simulink model "observerModel_GVS_MS"  (R2023b)
settings: Solver=ode15s  StartTime=0.0  StopTime=duration  MaxStep=0.02  RelTol=0.02  AbsTol=0.02  EnableMultiTasking=on
values from neighbouring files (symbols this model uses):
  beta1 = s(8)    [Observer_Analysis.m]
  beta2 = s(7)    [Observer_Analysis.m]
  delta_t = time(2) - time (1)    [Observer_Analysis.m]
  df = 1    [Observer_Analysis.m]
  f_oto = 2    [Observer_Analysis.m]
  f_scc = 2    [Observer_Analysis.m]
  f_visO = 0.2    [Observer_Analysis.m]
  f_visV = 2    [Observer_Analysis.m]
  f_visX = 2    [Observer_Analysis.m]
  GG0 = [0 0 -hypo]'    [Observer_Analysis.m]
  IrregDepol = tf(num,den)    [Observer_Analysis.m]
  IrregHyperpol = tf(num,den)    [Observer_Analysis.m]
  IrregSCC2Physical = inv(IrregSCCnf)    [Observer_Analysis.m]
  kaa = -3.2*[1 1 1]'    [Observer_Analysis.m]
  Kea = s(1)^(1/2)*[1 1 1]    [Observer_Analysis.m]
  Kef = s(3)^(1/2)*[1 1 1]    [Observer_Analysis.m]
  Kew = s(2)^(1/2)*[1 1 1]    [Observer_Analysis.m]
  Kfast = s(4)    [Observer_Analysis.m]
  kfg = 4*[1 1 1]'    [Observer_Analysis.m]
  kfw = 8*[1 1 1]'    [Observer_Analysis.m]
  kgvg = 5*[1 1 1]'    [Observer_Analysis.m]
  KLeft = 1-KRight    (= 0.5)    [Observer_Analysis.m]
  KReg = s2(2)    [Observer_Analysis.m]
  KRight = 0.5    [Observer_Analysis.m]
  KS = s2(1)*pi/180    [Observer_Analysis.m]
  kwg = 1*[1 1 1]'    [Observer_Analysis.m]
  kwvw = 10*[1 1 1]'    [Observer_Analysis.m]
  kww = 2.28*[1 1 1]'    [Observer_Analysis.m]
  kxdotva = 0.75*[1 1 1]'    [Observer_Analysis.m]
  kxvv = 0.1*[1 1 1]'    [Observer_Analysis.m]
  LeftSide_CurrentMult = s2(4)    [Observer_Analysis.m]
  ms_exp = s(6)    [Observer_Analysis.m]
  oto_a = 60*[1 1 1]'    [Observer_Analysis.m]
  oto_Ka = 1.3*[1 1 1]'    [Observer_Analysis.m]
  Q0 = [cos(E_angle/2) E(1)*sin(E_angle/2) E(2)*sin(E_angle/2) E(3)*sin(E_angle/2)]'    [Observer_Analysis.m]
  RegDepol = tf(num,den)    [Observer_Analysis.m]
  RegHyperpol = tf(num,den)    [Observer_Analysis.m]
  RegSCC2Physical = inv(RegSCCnf)    [Observer_Analysis.m]
  tau_a = tau_a_value*[1 1 1]'    [Observer_Analysis.m]
  tau_scc = tau_scc_value*[1 1 1]'    [Observer_Analysis.m]
  x_leak = 0.6    [Observer_Analysis.m]
  y_leak = 0.6    [Observer_Analysis.m]
  z_leak = 10    [Observer_Analysis.m]
(part 2 of 3)

== system observerModel_GVS_MS/Motion Sickness Dynamics/Oman 1 ==
  note: Ks = 5, Ts = 600sec, ns = 2
  note: Tf = 60sec, nf = 2
  note: if nf = 2, as Oman has it
  In1 : Inport
  Add1 : Sum
  Product : Product
  Transfer Fcn : TransferFcn  Numerator=[Kfast]  Denominator=[beta1^2 2*df*beta1 1]
  Transfer Fcn2 : TransferFcn  Denominator=[beta2^2 2*beta2 1]
  I(t) : Outport  VectorParamsAs1DForOutWhenUnconnected=off
  F(t) : Outport  Port=2  VectorParamsAs1DForOutWhenUnconnected=off
  S(t) : Outport  Port=3  VectorParamsAs1DForOutWhenUnconnected=off
  wires:
  Add1/1 -> I(t)/1  "I(t)"
  Transfer Fcn2/1 -> S(t)/1, Product/2, Add1/2  "S(t)"
  Transfer Fcn/1 -> Add1/1, F(t)/1  "F(t)"
  In1/1 -> Transfer Fcn2/1, Product/1
  Product/1 -> Transfer Fcn/1

== system observerModel_GVS_MS/Otoliths/X Graviceptor ==
  in_1 : Inport
  Adaptation : TransferFcn  Numerator=[oto_Ka(1)*oto_a(1) 1]  Denominator=[oto_a(1) 1]
  Low Pass Filter : TransferFcn  Denominator=[1/(2*pi*f_oto) 1]
  New Otolith model : TransferFcn  Numerator=[333 33.3]  Denominator="[0.08  5.016 1]"
  Scope{,1..3} (4 alike) : Scope
  X Graviceptor : TransferFcn  Numerator=[oto_Ka(1)*oto_a(1) 1]  Denominator=[oto_a(1)*1/(2*pi*f_oto) (1/(2*pi*f_oto)+oto_a(1)) 1]
  out_1 : Outport  InitialOutput=0
  wires:
  in_1/1 -> Low Pass Filter/1, X Graviceptor/1, Adaptation/1, New Otolith model/1
  Low Pass Filter/1 -> out_1/1, Scope2/1
  X Graviceptor/1 -> Scope/1
  Adaptation/1 -> Scope1/1
  New Otolith model/1 -> Scope3/1

== system observerModel_GVS_MS/Otoliths/Y Graviceptor ==
  in_1 : Inport
  Adaptation : TransferFcn  Numerator=[oto_Ka(2)*oto_a(2) 1]  Denominator=[oto_a(2) 1]
  Low Pass Filter : TransferFcn  Denominator=[1/(2*pi*f_oto) 1]
  New Otolith model : TransferFcn  Numerator=[333 33.3]  Denominator="[0.08  5.016 1]"
  Scope{,1..3} (4 alike) : Scope
  X Graviceptor : TransferFcn  Numerator=[oto_Ka(2)*oto_a(2) 1]  Denominator=[oto_a(2)*1/(2*pi*f_oto) (1/(2*pi*f_oto)+oto_a(2)) 1]
  out_1 : Outport  InitialOutput=0
  wires:
  in_1/1 -> Low Pass Filter/1, X Graviceptor/1, Adaptation/1, New Otolith model/1
  Low Pass Filter/1 -> out_1/1, Scope2/1
  X Graviceptor/1 -> Scope/1
  Adaptation/1 -> Scope1/1
  New Otolith model/1 -> Scope3/1

== system observerModel_GVS_MS/Otoliths/Z Graviceptor ==
  in_1 : Inport
  Adaptation : TransferFcn  Numerator=[oto_Ka(3)*oto_a(3) 1]  Denominator=[oto_a(3) 1]
  Low Pass Filter : TransferFcn  Denominator=[1/(2*pi*f_oto) 1]
  New Otolith model : TransferFcn  Numerator=[333 33.3]  Denominator="[0.08  5.016 1]"
  Scope{,1..3} (4 alike) : Scope
  X Graviceptor : TransferFcn  Numerator=[oto_Ka(3)*oto_a(3) 1]  Denominator=[oto_a(3)*1/(2*pi*f_oto) (1/(2*pi*f_oto)+oto_a(3)) 1]
  out_1 : Outport  InitialOutput=0
  wires:
  Low Pass Filter/1 -> out_1/1, Scope2/1
  X Graviceptor/1 -> Scope/1
  Adaptation/1 -> Scope1/1
  New Otolith model/1 -> Scope3/1
  in_1/1 -> Low Pass Filter/1, X Graviceptor/1, Adaptation/1, New Otolith model/1

== system observerModel_GVS_MS/Quaternion Rotator/Head to Limbic Angular Velocity Transform ==
  omega_head : Inport
  D_Cos : Inport  Port=2
  Gain : Gain  Gain=-1
  Product1 : Product  Multiplication=Matrix(*)  RndMeth=Zero
  Quaternion Integrator1 : Subsystem
  Quaternion to Direction Cosine1 : Subsystem
  Transform Axes : Subsystem
  Transpose : Math  Operator=transpose  SignedPower=on
  R_limbic : Outport
  wires:
  Quaternion Integrator1/1(q) -> Quaternion to Direction Cosine1/1(q)
  Quaternion to Direction Cosine1/1(D_Cos) -> R_limbic/1
  omega_head/1 -> Product1/2
  Transpose/1 -> Product1/1
  D_Cos/1 -> Transpose/1
  Product1/1 -> Transform Axes/1(limbic_cord)
  Transform Axes/1(VR_cord) -> Gain/1
  Gain/1 -> Quaternion Integrator1/1(omega_limbic)

== system observerModel_GVS_MS/Quaternion Rotator/Quaternion Integrator ==
  omega_head : Inport
  Demux1 : Demux
  Gain : Gain  Gain=1/delta_t
  Mux1 : Mux
  delta_q : Subsystem
  q0 : Integrator  InitialCondition=Q0(1)
  q1 : Integrator  InitialCondition=Q0(2)
  q2 : Integrator  InitialCondition=Q0(3)
  q3 : Integrator  InitialCondition=Q0(4)
  q : Outport
  wires:
  Demux1/1 -> q0/1
  q0/1 -> Mux1/1
  Demux1/2 -> q1/1
  q1/1 -> Mux1/2
  Demux1/3 -> q2/1
  q2/1 -> Mux1/3
  Demux1/4 -> q3/1
  q3/1 -> Mux1/4
  Mux1/1 -> delta_q/2(q), q/1
  Gain/1 -> Demux1/1
  delta_q/1(delta_q) -> Gain/1
  omega_head/1 -> delta_q/1(omega)

== system observerModel_GVS_MS/Quaternion Rotator/Quaternion to Direction Cosine ==
  note: A21
  q : Inport
  A1 : Subsystem
  A11 : Subsystem
  A12 : Subsystem
  A13 : Subsystem
  A22 : Subsystem
  A23 : Subsystem
  A31 : Subsystem
  A32 : Subsystem
  A33 : Subsystem
  Mux : Mux  Inputs=9
  Reshape (9) to [3x3] column-major : Reshape  OutputDimensionality=Customize  OutputDimensions=[3,3]
  D_Cos : Outport
  wires:
  A33/1(A33) -> Mux/9
  A32/1(A32) -> Mux/6
  A31/1(A31) -> Mux/3
  A23/1(A23) -> Mux/8
  A22/1(A22) -> Mux/5
  A13/1(A13) -> Mux/7
  A12/1(A12) -> Mux/4
  A11/1(A11) -> Mux/1
  q/1 -> A22/1(q), A1/1(q), A13/1(q), A12/1(q), A11/1(q), A23/1(q), A31/1(q), A32/1(q), A33/1(q)
  Reshape (9) to [3x3] column-major/1 -> D_Cos/1
  A1/1(A21) -> Mux/2
  Mux/1 -> Reshape (9) to [3x3] column-major/1

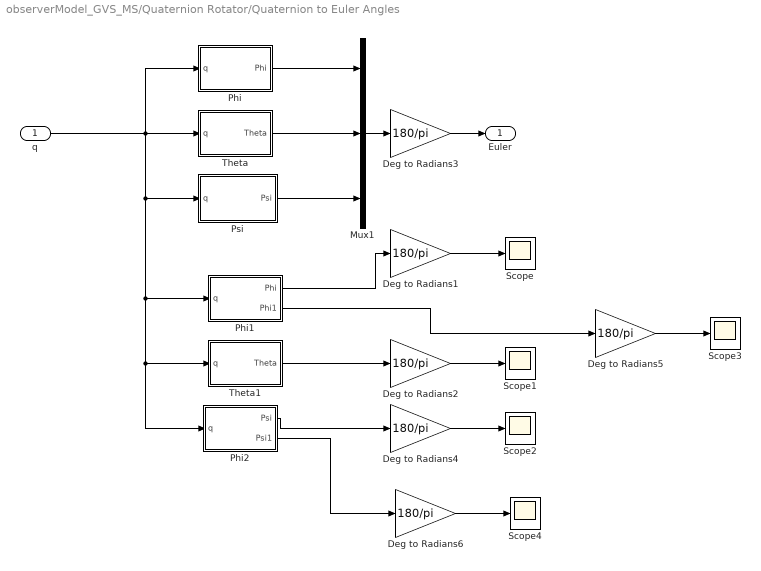
== system observerModel_GVS_MS/Quaternion Rotator/Quaternion to Euler Angles ==
  q : Inport
  Deg to Radians{1..6} (6 alike) : Gain  Gain=180/pi  SaturateOnIntegerOverflow=on  OutDataTypeStr=Inherit: Same as input  ParamDataTypeStr=Inherit: Same as input
  Mux1 : Mux  Inputs=3
  Phi : Subsystem
  Phi1 : Subsystem
  Phi2 : Subsystem
  Psi : Subsystem
  Scope{,1..4} (5 alike) : Scope
  Theta : Subsystem
  Theta1 : Subsystem
  Euler : Outport
  wires:
  Phi/1(Phi) -> Mux1/1
  Psi/1(Psi) -> Mux1/3
  Theta/1(Theta) -> Mux1/2
  q/1 -> Theta/1(q), Phi/1(q), Psi/1(q), Phi1/1(q), Theta1/1(q), Phi2/1(q)
  Mux1/1 -> Deg to Radians3/1
  Deg to Radians3/1 -> Euler/1
  Deg to Radians1/1 -> Scope/1
  Deg to Radians2/1 -> Scope1/1
  Deg to Radians4/1 -> Scope2/1
  Phi1/1(Phi) -> Deg to Radians1/1
  Theta1/1(Theta) -> Deg to Radians2/1
  Phi2/1(Psi) -> Deg to Radians4/1
  Deg to Radians5/1 -> Scope3/1
  Phi1/2(Phi1) -> Deg to Radians5/1
  Deg to Radians6/1 -> Scope4/1
  Phi2/2(Psi1) -> Deg to Radians6/1

== system observerModel_GVS_MS/Quaternion Rotator/Rotation ==
  D_Cos : Inport
  omega_rad : Inport  Port=2
  Azimuthal Integrator : Subsystem
  Ground Truth Gravity over time : FromWorkspace  VariableName=[t,G0]  ZeroCross=off
  Matrix Multiplication : Subsystem
  g : Outport
  azimuth : Outport  Port=2
  wires:
  D_Cos/1 -> Matrix Multiplication/1(D_Cos), Azimuthal Integrator/2(D_Cos)
  Matrix Multiplication/1(g) -> g/1, Azimuthal Integrator/1(g)
  omega_rad/1 -> Azimuthal Integrator/3(omega_rad)
  Azimuthal Integrator/1(azimuth) -> azimuth/1
  Ground Truth Gravity over time/1 -> Matrix Multiplication/2(G0)

== system observerModel_GVS_MS/Quaternion Rotator/Tilt & SVV ==
  g : Inport
  SVV Calculator : Subsystem
  Tilt Calculator : Subsystem
  Tilt : Outport
  SVV : Outport  Port=2
  wires:
  g/1 -> SVV Calculator/1(g), Tilt Calculator/1(g)
  Tilt Calculator/1(Tilt) -> Tilt/1
  SVV Calculator/1(SVV) -> SVV/1

== system observerModel_GVS_MS/Quaternion Rotator2/Head to Limbic Angular Velocity Transform Rotation Matrix ==
  omega_est : Inport
  D_Cos : Inport  Port=2
  Gain : Gain  Gain=-1
  Product1 : Product  Multiplication=Matrix(*)  RndMeth=Zero
  Quaternion Integrator1 : Subsystem
  Quaternion to Direction Cosine1 : Subsystem
  Transform Axes : Subsystem
  Transpose : Math  Operator=transpose  SignedPower=on
  R_limbic_est : Outport
  wires:
  Quaternion Integrator1/1(q) -> Quaternion to Direction Cosine1/1(q)
  Quaternion to Direction Cosine1/1(D_Cos) -> R_limbic_est/1
  omega_est/1 -> Product1/2
  Transpose/1 -> Product1/1
  D_Cos/1 -> Transpose/1
  Product1/1 -> Transform Axes/1(limbic_cord)
  Transform Axes/1(VR_cord) -> Gain/1
  Gain/1 -> Quaternion Integrator1/1(omega_limbic)

== system observerModel_GVS_MS/Quaternion Rotator2/Quaternion Integrator ==
  omega_rad_est : Inport
  Demux1 : Demux
  Gain : Gain  Gain=1/delta_t
  Mux1 : Mux
  delta_q : Subsystem
  q0 : Integrator  InitialCondition=Q0(1)
  q1 : Integrator  InitialCondition=Q0(2)
  q2 : Integrator  InitialCondition=Q0(3)
  q3 : Integrator  InitialCondition=Q0(4)
  q : Outport
  wires:
  Demux1/1 -> q0/1
  q0/1 -> Mux1/1
  Demux1/2 -> q1/1
  q1/1 -> Mux1/2
  Demux1/3 -> q2/1
  q2/1 -> Mux1/3
  Demux1/4 -> q3/1
  q3/1 -> Mux1/4
  Mux1/1 -> delta_q/2(q), q/1
  Gain/1 -> Demux1/1
  delta_q/1(delta_q) -> Gain/1
  omega_rad_est/1 -> delta_q/1(omega)

== system observerModel_GVS_MS/Quaternion Rotator2/Quaternion to Direction Cosine ==
  note: A21
  q : Inport
  A1 : Subsystem
  A11 : Subsystem
  A12 : Subsystem
  A13 : Subsystem
  A22 : Subsystem
  A23 : Subsystem
  A31 : Subsystem
  A32 : Subsystem
  A33 : Subsystem
  Mux : Mux  Inputs=9
  Reshape (9) to [3x3] column-major : Reshape  OutputDimensionality=Customize  OutputDimensions=[3,3]
  D_Cos : Outport
  wires:
  A33/1(A33) -> Mux/9
  A32/1(A32) -> Mux/6
  A31/1(A31) -> Mux/3
  A23/1(A23) -> Mux/8
  A22/1(A22) -> Mux/5
  A13/1(A13) -> Mux/7
  A12/1(A12) -> Mux/4
  A11/1(A11) -> Mux/1
  q/1 -> A22/1(q), A1/1(q), A13/1(q), A12/1(q), A11/1(q), A23/1(q), A31/1(q), A32/1(q), A33/1(q)
  Reshape (9) to [3x3] column-major/1 -> D_Cos/1
  A1/1(A21) -> Mux/2
  Mux/1 -> Reshape (9) to [3x3] column-major/1

== system observerModel_GVS_MS/Quaternion Rotator2/Quaternion to Euler Angles ==
  q : Inport
  Deg to Radians3 : Gain  Gain=180/pi  SaturateOnIntegerOverflow=on  OutDataTypeStr=Inherit: Same as input  ParamDataTypeStr=Inherit: Same as input
  Mux1 : Mux  Inputs=3
  Phi : Subsystem
  Psi : Subsystem
  Theta : Subsystem
  Euler : Outport
  wires:
  Phi/1(Phi) -> Mux1/1
  Psi/1(Psi) -> Mux1/3
  Theta/1(Theta) -> Mux1/2
  q/1 -> Phi/1(q), Theta/1(q), Psi/1(q)
  Mux1/1 -> Deg to Radians3/1
  Deg to Radians3/1 -> Euler/1

== system observerModel_GVS_MS/Quaternion Rotator2/Rotation ==
  D_Cos : Inport
  omega_rad : Inport  Port=2
  Azimuthal Integrator : Subsystem
  Hypo Gravity State : Constant  Value=GG0  VectorParams1D=off
  Matrix Multiplication : Subsystem
  g : Outport
  azimuth : Outport  Port=2
  wires:
  Hypo Gravity State/1 -> Matrix Multiplication/2(GG0)
  D_Cos/1 -> Matrix Multiplication/1(D_Cos), Azimuthal Integrator/2(D_Cos)
  Matrix Multiplication/1(g) -> g/1, Azimuthal Integrator/1(g)
  omega_rad/1 -> Azimuthal Integrator/3(omega_rad)
  Azimuthal Integrator/1(azimuth) -> azimuth/1

== system observerModel_GVS_MS/Quaternion Rotator2/Tilt & SVV ==
  g : Inport
  SVV Calculator : Subsystem
  Tilt Calculator : Subsystem
  Tilt : Outport
  SVV : Outport  Port=2
  wires:
  g/1 -> Tilt Calculator/1(g), SVV Calculator/1(g)
  Tilt Calculator/1(Tilt) -> Tilt/1
  SVV Calculator/1(SVV) -> SVV/1

== system observerModel_GVS_MS/SCC GVS /Left Irregular Hyper//Depol  ==
  In1 : Inport
  If : If
  If Action Subsystem : Subsystem  TreatAsAtomicUnit=on
  If Action Subsystem1 : Subsystem  TreatAsAtomicUnit=on
  Merge : Merge
  Out1 : Outport
  wires:
  In1/1 -> If Action Subsystem1/1(In1), If Action Subsystem/1(In1), If/1
  Merge/1 -> Out1/1
  If/1 -> If Action Subsystem/Action
  If Action Subsystem/1(Out1) -> Merge/1
  If Action Subsystem1/1(Out1) -> Merge/2
  If/2 -> If Action Subsystem1/Action

== system observerModel_GVS_MS/SCC GVS /Left Regular Hyper//Depol ==
  In1 : Inport
  If : If
  If Action Subsystem : Subsystem  TreatAsAtomicUnit=on
  If Action Subsystem1 : Subsystem  TreatAsAtomicUnit=on
  Merge : Merge
  Out1 : Outport
  wires:
  In1/1 -> If Action Subsystem1/1(In1), If Action Subsystem/1(In1), If/1
  Merge/1 -> Out1/1
  If/1 -> If Action Subsystem/Action
  If Action Subsystem/1(Out1) -> Merge/1
  If Action Subsystem1/1(Out1) -> Merge/2
  If/2 -> If Action Subsystem1/Action

== system observerModel_GVS_MS/SCC GVS /Right Irregular Hyper//Depol  ==
  In1 : Inport
  If : If
  If Action Subsystem : Subsystem  TreatAsAtomicUnit=on
  If Action Subsystem1 : Subsystem  TreatAsAtomicUnit=on
  Merge : Merge
  Out1 : Outport
  wires:
  In1/1 -> If Action Subsystem1/1(In1), If Action Subsystem/1(In1), If/1
  Merge/1 -> Out1/1
  If/1 -> If Action Subsystem/Action
  If Action Subsystem/1(Out1) -> Merge/1
  If Action Subsystem1/1(Out1) -> Merge/2
  If/2 -> If Action Subsystem1/Action

== system observerModel_GVS_MS/SCC GVS /Right Regular Hyper//Depol  ==
  In1 : Inport
  If : If
  If Action Subsystem : Subsystem  TreatAsAtomicUnit=on
  If Action Subsystem1 : Subsystem  TreatAsAtomicUnit=on
  Merge : Merge
  Out1 : Outport
  wires:
  In1/1 -> If Action Subsystem1/1(In1), If Action Subsystem/1(In1), If/1
  Merge/1 -> Out1/1
  If/1 -> If Action Subsystem/Action
  If Action Subsystem/1(Out1) -> Merge/1
  If Action Subsystem1/1(Out1) -> Merge/2
  If/2 -> If Action Subsystem1/Action

== system observerModel_GVS_MS/Subsystem/Matrix Multiplication ==
  D_Cos : Inport
  a_world : Inport  Port=2
  Demux : Demux  Outputs=3
      settings: DisplayOption=none
  Mux : Mux  Inputs=3
  Product : Product  Multiplication=Matrix(*)  RndMeth=Zero
  a_head : Outport
  wires:
  Product/1 -> Demux/1
  Demux/1 -> Mux/1
  Demux/2 -> Mux/2
  Demux/3 -> Mux/3
  D_Cos/1 -> Product/1
  Mux/1 -> a_head/1
  a_world/1 -> Product/2

== system observerModel_GVS_MS/Subsystem13/Matrix Multiplication ==
  D_Cos : Inport
  a_esr_head : Inport  Port=2
  Demux : Demux  Outputs=3
      settings: DisplayOption=none
  Math Function : Math  Operator=transpose  SignedPower=on
  Mux : Mux  Inputs=3
  Product : Product  Multiplication=Matrix(*)  RndMeth=Zero
  a_est_world : Outport
  wires:
  Product/1 -> Demux/1
  Demux/1 -> Mux/1
  Demux/2 -> Mux/2
  Demux/3 -> Mux/3
  D_Cos/1 -> Math Function/1
  Mux/1 -> a_est_world/1
  a_esr_head/1 -> Product/2
  Math Function/1 -> Product/1

== system observerModel_GVS_MS/Subsystem2/Matrix Multiplication ==
  D_Cos : Inport
  a_est_head : Inport  Port=2
  Demux : Demux  Outputs=3
      settings: DisplayOption=none
  Math Function : Math  Operator=transpose  SignedPower=on
  Mux : Mux  Inputs=3
  Product : Product  Multiplication=Matrix(*)  RndMeth=Zero
  a_est_world : Outport
  wires:
  Product/1 -> Demux/1
  Demux/1 -> Mux/1
  Demux/2 -> Mux/2
  Demux/3 -> Mux/3
  D_Cos/1 -> Math Function/1
  Mux/1 -> a_est_world/1
  a_est_head/1 -> Product/2
  Math Function/1 -> Product/1

== system observerModel_GVS_MS/Subsystem3/Subsystem3 ==
  In1 : Inport
  Matrix Multiplication : Subsystem
  Out1 : Outport
  wires:
  [D_Cos] -> Matrix Multiplication/1(D_Cos)
  Matrix Multiplication/1(a_head) -> Out1/1
  In1/1 -> Matrix Multiplication/2(a_world)

== system observerModel_GVS_MS/Subsystem3/Subsystem4 ==
  In1 : Inport
  Matrix Multiplication : Subsystem
  Out1 : Outport
  wires:
  [D_Cos_est] -> Matrix Multiplication/1(D_Cos)
  Matrix Multiplication/1(a_est_world) -> Out1/1
  In1/1 -> Matrix Multiplication/2(a_esr_head)

== system observerModel_GVS_MS/Subsystem5/Subsystem3 ==
  In1 : Inport
  Matrix Multiplication : Subsystem
  Out1 : Outport
  wires:
  [D_Cos] -> Matrix Multiplication/1(D_Cos)
  Matrix Multiplication/1(a_head) -> Out1/1
  In1/1 -> Matrix Multiplication/2(a_world)

== system observerModel_GVS_MS/Subsystem5/Subsystem4 ==
  In1 : Inport
  Matrix Multiplication : Subsystem
  Out1 : Outport
  wires:
  [D_Cos_est] -> Matrix Multiplication/1(D_Cos)
  Matrix Multiplication/1(a_est_world) -> Out1/1
  In1/1 -> Matrix Multiplication/2(a_esr_head)

== system observerModel_GVS_MS/Subsystem6/Matrix Multiplication ==
  D_Cos : Inport
  a_world : Inport  Port=2
  Demux : Demux  Outputs=3
      settings: DisplayOption=none
  Mux : Mux  Inputs=3
  Product : Product  Multiplication=Matrix(*)  RndMeth=Zero
  a_head : Outport
  wires:
  Product/1 -> Demux/1
  Demux/1 -> Mux/1
  Demux/2 -> Mux/2
  Demux/3 -> Mux/3
  D_Cos/1 -> Product/1
  Mux/1 -> a_head/1
  a_world/1 -> Product/2

== system observerModel_GVS_MS/To VR (actual)/Limbic to VR Displacement ==
  Limbic Displacement : Inport
  Scale Gain : Gain  Gain=30
  Transform Axes Translation : Subsystem
  VR Displacement : Outport
  wires:
  Transform Axes Translation/1(VR_cord) -> Scale Gain/1
  Scale Gain/1 -> VR Displacement/1
  Limbic Displacement/1 -> Transform Axes Translation/1(head_cord)

== system observerModel_GVS_MS/To VR (est)/Limbic to VR Estimated Displacement ==
  Limbic Est Displacement : Inport
  Scale Gain : Gain  Gain=30
  Transform Axes Translation Est : Subsystem
  VR Est Displacement : Outport
  wires:
  Transform Axes Translation Est/1(VR_cord) -> Scale Gain/1
  Scale Gain/1 -> VR Est Displacement/1
  Limbic Est Displacement/1 -> Transform Axes Translation Est/1(head_cord)

== system observerModel_GVS_MS/Quaternion Rotator/Head to Limbic Angular Velocity Transform/Quaternion Integrator1 ==
  omega_limbic : Inport
  Demux1 : Demux
  Gain : Gain  Gain=1/delta_t
  Mux1 : Mux
  delta_q : Subsystem
  q0 : Integrator  InitialCondition=Q0(1)
  q1 : Integrator  InitialCondition=Q0(3)
  q2 : Integrator  InitialCondition=Q0(4)
  q3 : Integrator  InitialCondition=Q0(2)
  q : Outport
  wires:
  Demux1/1 -> q0/1
  Demux1/2 -> q1/1
  Demux1/3 -> q2/1
  Demux1/4 -> q3/1
  Mux1/1 -> delta_q/2(q), q/1
  Gain/1 -> Demux1/1
  delta_q/1(delta_q) -> Gain/1
  omega_limbic/1 -> delta_q/1(omega)
  q0/1 -> Mux1/1
  q2/1 -> Mux1/3
  q3/1 -> Mux1/4
  q1/1 -> Mux1/2

== system observerModel_GVS_MS/Quaternion Rotator/Head to Limbic Angular Velocity Transform/Quaternion to Direction Cosine1 ==
  note: A21
  q : Inport
  A1 : Subsystem
  A11 : Subsystem
  A12 : Subsystem
  A13 : Subsystem
  A22 : Subsystem
  A23 : Subsystem
  A31 : Subsystem
  A32 : Subsystem
  A33 : Subsystem
  Mux : Mux  Inputs=9
  Reshape (9) to [3x3] column-major : Reshape  OutputDimensionality=Customize  OutputDimensions=[3,3]
  D_Cos : Outport
  wires:
  A33/1(A33) -> Mux/9
  A32/1(A32) -> Mux/6
  A31/1(A31) -> Mux/3
  A23/1(A23) -> Mux/8
  A22/1(A22) -> Mux/5
  A13/1(A13) -> Mux/7
  A12/1(A12) -> Mux/4
  A11/1(A11) -> Mux/1
  q/1 -> A22/1(q), A1/1(q), A13/1(q), A12/1(q), A11/1(q), A23/1(q), A31/1(q), A32/1(q), A33/1(q)
  Reshape (9) to [3x3] column-major/1 -> D_Cos/1
  A1/1(A21) -> Mux/2
  Mux/1 -> Reshape (9) to [3x3] column-major/1

== system observerModel_GVS_MS/Quaternion Rotator/Head to Limbic Angular Velocity Transform/Transform Axes ==
  limbic_cord : Inport
  Demux2 : Demux  Outputs=3
  Mux2 : Mux  Inputs=3
  VR_cord : Outport
  wires:
  limbic_cord/1 -> Demux2/1
  Mux2/1 -> VR_cord/1
  Demux2/3 -> Mux2/2
  Demux2/1 -> Mux2/3
  Demux2/2 -> Mux2/1

== system observerModel_GVS_MS/Quaternion Rotator/Quaternion Integrator/delta_q ==
  omega : Inport
  q : Inport  Port=2
  C : Subsystem
  Constant : Constant  Value=delta_t
  K : Subsystem
  Product : Product  RndMeth=Zero
  Product1 : Product  RndMeth=Zero
  Product2 : Product  RndMeth=Zero
  Sum : Sum
  Z : Subsystem
  delta_q : Outport
  wires:
  q/1 -> C/2(q), Z/1(q), Product1/1
  Z/1(z) -> Product/1
  Product/1 -> Product1/2
  Product1/1 -> Sum/2
  C/1(C) -> Sum/1
  Sum/1 -> Product2/2
  Constant/1 -> Product2/1
  omega/1 -> C/1(omega)
  Product2/1 -> delta_q/1
  K/1(K) -> Product/2

== system observerModel_GVS_MS/Quaternion Rotator/Quaternion to Direction Cosine/A1 ==
  q : Inport
  Demux : Demux
  Gain : Gain  Gain=2
  Product : Product  RndMeth=Zero
  Product1 : Product  RndMeth=Zero
  Sum : Sum  Inputs=+-
  A21 : Outport
  wires:
  q/1 -> Demux/1
  Sum/1 -> Gain/1
  Gain/1 -> A21/1
  Product/1 -> Sum/1
  Product1/1 -> Sum/2
  Demux/2 -> Product/1
  Demux/3 -> Product/2
  Demux/1 -> Product1/1
  Demux/4 -> Product1/2

== system observerModel_GVS_MS/Quaternion Rotator/Quaternion to Direction Cosine/A11 ==
  q : Inport
  Demux : Demux
  Product{,1..3} (4 alike) : Product  RndMeth=Zero
  Sum : Sum  Inputs=++--
  A11 : Outport
  wires:
  Demux/1 -> Product/1, Product/2
  Demux/2 -> Product1/1, Product1/2
  Demux/3 -> Product2/1, Product2/2
  Demux/4 -> Product3/1, Product3/2
  Product/1 -> Sum/1
  Product1/1 -> Sum/2
  Product2/1 -> Sum/3
  Product3/1 -> Sum/4
  q/1 -> Demux/1
  Sum/1 -> A11/1

== system observerModel_GVS_MS/Quaternion Rotator/Quaternion to Direction Cosine/A12 ==
  q : Inport
  Demux : Demux
  Gain : Gain  Gain=2
  Product : Product  RndMeth=Zero
  Product1 : Product  RndMeth=Zero
  Sum : Sum
  A12 : Outport
  wires:
  q/1 -> Demux/1
  Sum/1 -> Gain/1
  Gain/1 -> A12/1
  Demux/2 -> Product/1
  Demux/3 -> Product/2
  Demux/1 -> Product1/1
  Demux/4 -> Product1/2
  Product/1 -> Sum/1
  Product1/1 -> Sum/2

== system observerModel_GVS_MS/Quaternion Rotator/Quaternion to Direction Cosine/A13 ==
  q : Inport
  Demux : Demux
  Gain : Gain  Gain=2
  Product : Product  RndMeth=Zero
  Product1 : Product  RndMeth=Zero
  Sum : Sum  Inputs=+-
  A13 : Outport
  wires:
  q/1 -> Demux/1
  Sum/1 -> Gain/1
  Gain/1 -> A13/1
  Product/1 -> Sum/1
  Product1/1 -> Sum/2
  Demux/2 -> Product/1
  Demux/4 -> Product/2
  Demux/1 -> Product1/1
  Demux/3 -> Product1/2

== system observerModel_GVS_MS/Quaternion Rotator/Quaternion to Direction Cosine/A22 ==
  q : Inport
  Demux : Demux
  Product{,1..3} (4 alike) : Product  RndMeth=Zero
  Sum : Sum  Inputs=+-+-
  A22 : Outport
  wires:
  Demux/1 -> Product/1, Product/2
  Demux/2 -> Product1/1, Product1/2
  Demux/3 -> Product2/1, Product2/2
  Demux/4 -> Product3/1, Product3/2
  Product/1 -> Sum/1
  Product1/1 -> Sum/2
  Product2/1 -> Sum/3
  Product3/1 -> Sum/4
  q/1 -> Demux/1
  Sum/1 -> A22/1

== system observerModel_GVS_MS/Quaternion Rotator/Quaternion to Direction Cosine/A23 ==
  q : Inport
  Demux : Demux
  Gain : Gain  Gain=2
  Product : Product  RndMeth=Zero
  Product1 : Product  RndMeth=Zero
  Sum : Sum
  A23 : Outport
  wires:
  q/1 -> Demux/1
  Sum/1 -> Gain/1
  Gain/1 -> A23/1
  Product/1 -> Sum/1
  Product1/1 -> Sum/2
  Demux/3 -> Product1/1
  Demux/4 -> Product1/2
  Demux/1 -> Product/1
  Demux/2 -> Product/2

== system observerModel_GVS_MS/Quaternion Rotator/Quaternion to Direction Cosine/A31 ==
  q : Inport
  Demux : Demux
  Gain : Gain  Gain=2
  Product : Product  RndMeth=Zero
  Product1 : Product  RndMeth=Zero
  Sum : Sum
  A31 : Outport
  wires:
  q/1 -> Demux/1
  Sum/1 -> Gain/1
  Gain/1 -> A31/1
  Product/1 -> Sum/1
  Product1/1 -> Sum/2
  Demux/1 -> Product/1
  Demux/3 -> Product/2
  Demux/2 -> Product1/1
  Demux/4 -> Product1/2

== system observerModel_GVS_MS/Quaternion Rotator/Quaternion to Direction Cosine/A32 ==
  q : Inport
  Demux : Demux
  Gain : Gain  Gain=2
  Product : Product  RndMeth=Zero
  Product1 : Product  RndMeth=Zero
  Sum : Sum  Inputs=+-
  A32 : Outport
  wires:
  q/1 -> Demux/1
  Sum/1 -> Gain/1
  Gain/1 -> A32/1
  Product/1 -> Sum/1
  Product1/1 -> Sum/2
  Demux/3 -> Product/1
  Demux/4 -> Product/2
  Demux/1 -> Product1/1
  Demux/2 -> Product1/2

== system observerModel_GVS_MS/Quaternion Rotator/Quaternion to Direction Cosine/A33 ==
  q : Inport
  Demux : Demux
  Product{,1..3} (4 alike) : Product  RndMeth=Zero
  Sum : Sum  Inputs=+--+
  A33 : Outport
  wires:
  Demux/1 -> Product/1, Product/2
  Demux/2 -> Product1/1, Product1/2
  Demux/3 -> Product2/1, Product2/2
  Demux/4 -> Product3/1, Product3/2
  Product/1 -> Sum/1
  Product1/1 -> Sum/2
  Product2/1 -> Sum/3
  Product3/1 -> Sum/4
  q/1 -> Demux/1
  Sum/1 -> A33/1

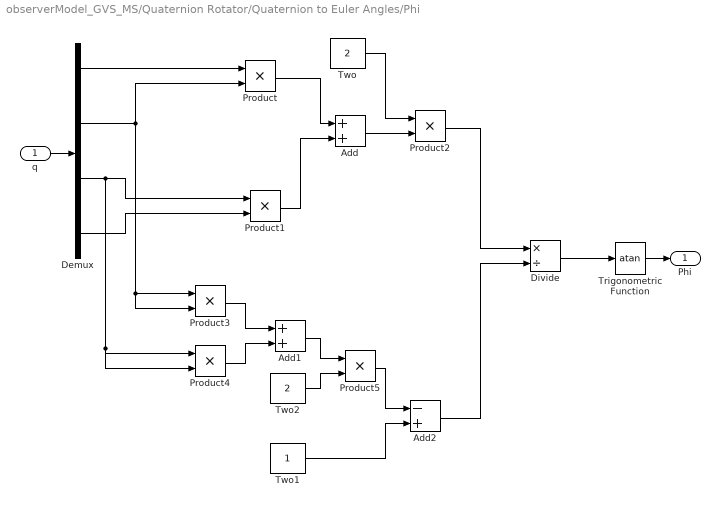
== system observerModel_GVS_MS/Quaternion Rotator/Quaternion to Euler Angles/Phi ==
  q : Inport
  Add : Sum
  Add1 : Sum
  Add2 : Sum  Inputs=-+
  Demux : Demux
  Divide : Product  Inputs=*/
  Product{,1..5} (6 alike) : Product  RndMeth=Zero
  Trigonometric Function : Trigonometry  Operator=atan
  Two : Constant  Value=2  VectorParams1D=off
  Two1 : Constant  VectorParams1D=off
  Two2 : Constant  Value=2  VectorParams1D=off
  Phi : Outport
  wires:
  Demux/1 -> Product/1
  Demux/2 -> Product/2, Product3/1, Product3/2
  Product/1 -> Add/1
  Demux/4 -> Product1/2
  Demux/3 -> Product1/1, Product4/1, Product4/2
  Product1/1 -> Add/2
  Add/1 -> Product2/2
  Two/1 -> Product2/1
  Product3/1 -> Add1/1
  Product4/1 -> Add1/2
  Add1/1 -> Product5/1
  Two2/1 -> Product5/2
  Product5/1 -> Add2/1
  Two1/1 -> Add2/2
  Product2/1 -> Divide/1
  Add2/1 -> Divide/2
  Divide/1 -> Trigonometric Function/1
  q/1 -> Demux/1
  Trigonometric Function/1 -> Phi/1

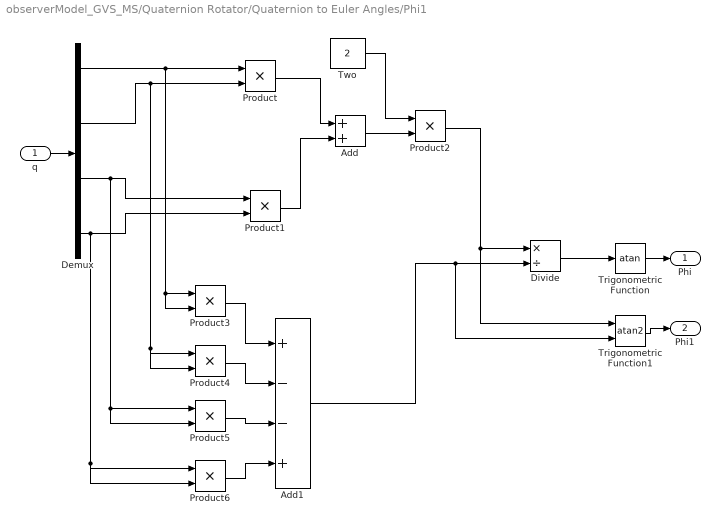
== system observerModel_GVS_MS/Quaternion Rotator/Quaternion to Euler Angles/Phi1 ==
  q : Inport
  Add : Sum
  Add1 : Sum  Inputs=+--+
  Demux : Demux
  Divide : Product  Inputs=*/
  Product{,1..6} (7 alike) : Product  RndMeth=Zero
  Trigonometric Function : Trigonometry  Operator=atan
  Trigonometric Function1 : Trigonometry  Operator=atan2
  Two : Constant  Value=2  VectorParams1D=off
  Phi : Outport
  Phi1 : Outport  Port=2
  wires:
  Demux/1 -> Product/1, Product3/1, Product3/2
  Demux/2 -> Product/2, Product4/1, Product4/2
  Product/1 -> Add/1
  Demux/4 -> Product1/2, Product6/1, Product6/2
  Demux/3 -> Product1/1, Product5/1, Product5/2
  Product1/1 -> Add/2
  Add/1 -> Product2/2
  Two/1 -> Product2/1
  Product3/1 -> Add1/1
  Product4/1 -> Add1/2
  Product2/1 -> Divide/1, Trigonometric Function1/1
  Divide/1 -> Trigonometric Function/1
  q/1 -> Demux/1
  Trigonometric Function/1 -> Phi/1
  Product5/1 -> Add1/3
  Product6/1 -> Add1/4
  Add1/1 -> Divide/2, Trigonometric Function1/2
  Trigonometric Function1/1 -> Phi1/1

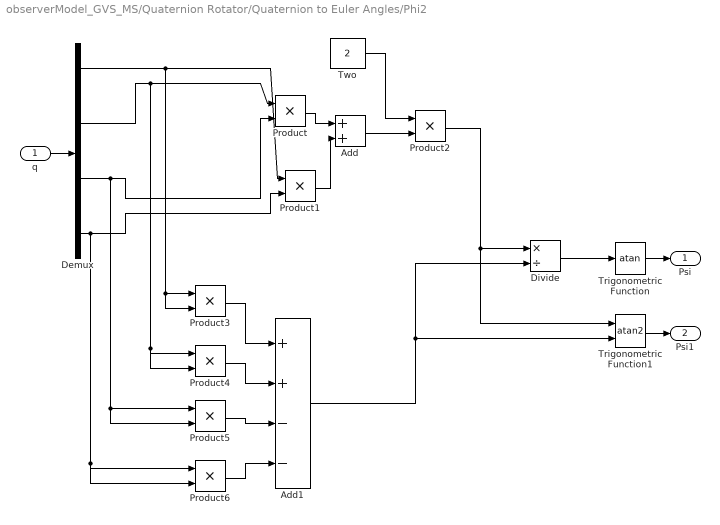
== system observerModel_GVS_MS/Quaternion Rotator/Quaternion to Euler Angles/Phi2 ==
  q : Inport
  Add : Sum
  Add1 : Sum  Inputs=++--
  Demux : Demux
  Divide : Product  Inputs=*/
  Product{,1..6} (7 alike) : Product  RndMeth=Zero
  Trigonometric Function : Trigonometry  Operator=atan
  Trigonometric Function1 : Trigonometry  Operator=atan2
  Two : Constant  Value=2  VectorParams1D=off
  Psi : Outport
  Psi1 : Outport  Port=2
  wires:
  Demux/1 -> Product3/1, Product3/2, Product1/1
  Demux/2 -> Product4/1, Product4/2, Product/1
  Demux/4 -> Product6/1, Product6/2, Product1/2
  Demux/3 -> Product5/1, Product5/2, Product/2
  Add/1 -> Product2/2
  Two/1 -> Product2/1
  Product3/1 -> Add1/1
  Product4/1 -> Add1/2
  Product2/1 -> Divide/1, Trigonometric Function1/1
  Divide/1 -> Trigonometric Function/1
  q/1 -> Demux/1
  Trigonometric Function/1 -> Psi/1
  Product5/1 -> Add1/3
  Product6/1 -> Add1/4
  Add1/1 -> Divide/2, Trigonometric Function1/2
  Product1/1 -> Add/2
  Product/1 -> Add/1
  Trigonometric Function1/1 -> Psi1/1

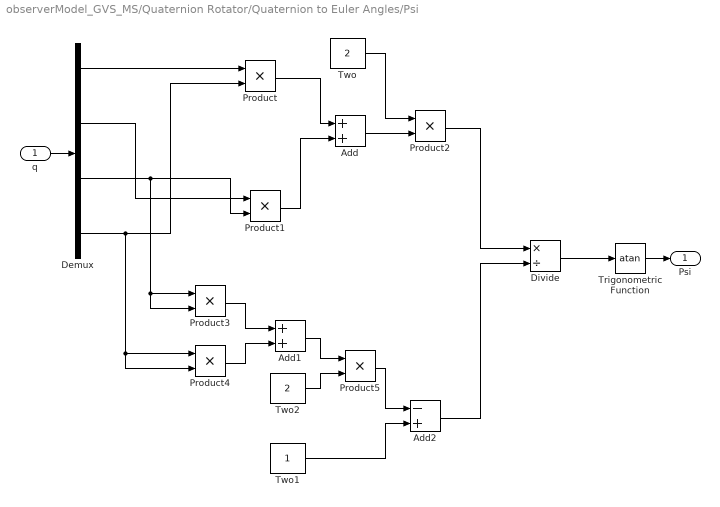
== system observerModel_GVS_MS/Quaternion Rotator/Quaternion to Euler Angles/Psi ==
  q : Inport
  Add : Sum
  Add1 : Sum
  Add2 : Sum  Inputs=-+
  Demux : Demux
  Divide : Product  Inputs=*/
  Product{,1..5} (6 alike) : Product  RndMeth=Zero
  Trigonometric Function : Trigonometry  Operator=atan
  Two : Constant  Value=2  VectorParams1D=off
  Two1 : Constant  VectorParams1D=off
  Two2 : Constant  Value=2  VectorParams1D=off
  Psi : Outport
  wires:
  Demux/2 -> Product1/1
  Product/1 -> Add/1
  Demux/4 -> Product4/1, Product4/2, Product/2
  Product1/1 -> Add/2
  Add/1 -> Product2/2
  Two/1 -> Product2/1
  Product3/1 -> Add1/1
  Product4/1 -> Add1/2
  Add1/1 -> Product5/1
  Two2/1 -> Product5/2
  Product5/1 -> Add2/1
  Two1/1 -> Add2/2
  Product2/1 -> Divide/1
  Add2/1 -> Divide/2
  Divide/1 -> Trigonometric Function/1
  q/1 -> Demux/1
  Trigonometric Function/1 -> Psi/1
  Demux/1 -> Product/1
  Demux/3 -> Product1/2, Product3/1, Product3/2

== system observerModel_GVS_MS/Quaternion Rotator/Quaternion to Euler Angles/Theta ==
  q : Inport
  Add : Sum  Inputs=+-
  Demux : Demux
  Product : Product  RndMeth=Zero
  Product1 : Product  RndMeth=Zero
  Product2 : Product  RndMeth=Zero
  Trigonometric Function : Trigonometry  Operator=asin
  Two : Constant  Value=2  VectorParams1D=off
  Theta : Outport
  wires:
  Demux/1 -> Product/1
  Product/1 -> Add/1
  Demux/4 -> Product1/2
  Product1/1 -> Add/2
  Add/1 -> Product2/2
  Two/1 -> Product2/1
  q/1 -> Demux/1
  Trigonometric Function/1 -> Theta/1
  Product2/1 -> Trigonometric Function/1
  Demux/3 -> Product/2
  Demux/2 -> Product1/1

== system observerModel_GVS_MS/Quaternion Rotator/Quaternion to Euler Angles/Theta1 ==
  q : Inport
  Add : Sum  Inputs=+-
  Demux : Demux
  Product : Product  RndMeth=Zero
  Product1 : Product  RndMeth=Zero
  Product2 : Product  RndMeth=Zero
  Trigonometric Function : Trigonometry  Operator=asin
  Two : Constant  Value=2  VectorParams1D=off
  Theta : Outport
  wires:
  Demux/1 -> Product/1
  Product/1 -> Add/1
  Demux/4 -> Product1/2
  Product1/1 -> Add/2
  Add/1 -> Product2/2
  Two/1 -> Product2/1
  q/1 -> Demux/1
  Trigonometric Function/1 -> Theta/1
  Product2/1 -> Trigonometric Function/1
  Demux/3 -> Product/2
  Demux/2 -> Product1/1

== system observerModel_GVS_MS/Quaternion Rotator/Rotation/Azimuthal Integrator ==
  g : Inport
  D_Cos : Inport  Port=2
  omega_rad : Inport  Port=3
  Dot Product : DotProduct  OutDataTypeStr=Inherit: Inherit via internal rule
  Gain : Gain  Gain=180/3.14159
  Integrator : Integrator
  Matrix Multiplication1 : Subsystem
  Scope1 : Scope
  azimuth : Outport
  wires:
  Matrix Multiplication1/1(omega_rad') -> Dot Product/2
  Dot Product/1 -> Gain/1, Integrator/1
  Gain/1 -> Scope1/1
  Integrator/1 -> azimuth/1
  g/1 -> Dot Product/1
  D_Cos/1 -> Matrix Multiplication1/1(D_Cos)
  omega_rad/1 -> Matrix Multiplication1/2(omega_rad)

== system observerModel_GVS_MS/Quaternion Rotator/Rotation/Matrix Multiplication ==
  D_Cos : Inport
  G0 : Inport  Port=2
  Demux : Demux  Outputs=3
      settings: DisplayOption=none
  Mux : Mux  Inputs=3
  Product : Product  Multiplication=Matrix(*)  RndMeth=Zero
  g : Outport
  wires:
  Product/1 -> Demux/1
  Demux/1 -> Mux/1
  Demux/2 -> Mux/2
  Demux/3 -> Mux/3
  D_Cos/1 -> Product/1
  Mux/1 -> g/1
  G0/1 -> Product/2

== system observerModel_GVS_MS/Quaternion Rotator/Tilt & SVV/SVV Calculator ==
  g : Inport
  Demux : Demux  Outputs=3
  Divide : Product  Inputs=*/
  Terminator : Terminator
  Trigonometric Function : Trigonometry  Operator=atan
  SVV : Outport
  wires:
  Divide/1 -> Trigonometric Function/1
  g/1 -> Demux/1
  Trigonometric Function/1 -> SVV/1
  Demux/2 -> Divide/1
  Demux/3 -> Divide/2
  Demux/1 -> Terminator/1

== system observerModel_GVS_MS/Quaternion Rotator/Tilt & SVV/Tilt Calculator ==
  g : Inport
  Add : Sum  Inputs=+++
  Demux : Demux  Outputs=3
  Divide : Product  Inputs=*/
  Math Function : Math  Operator=sqrt  SignedPower=on
  Product{,1..3} (4 alike) : Product  RndMeth=Zero
  Trigonometric Function : Trigonometry  Operator=acos  OutputSignalType=real
  Two : Constant  Value=-1  VectorParams1D=off
  Tilt : Outport
  wires:
  Product/1 -> Add/1
  Product1/1 -> Add/2
  Divide/1 -> Trigonometric Function/1
  g/1 -> Demux/1
  Product2/1 -> Add/3
  Demux/1 -> Product/1, Product/2
  Demux/2 -> Product1/2, Product1/1
  Demux/3 -> Product2/2, Product2/1, Product3/1
  Add/1 -> Math Function/1
  Two/1 -> Product3/2
  Math Function/1 -> Divide/2
  Product3/1 -> Divide/1
  Trigonometric Function/1 -> Tilt/1

== system observerModel_GVS_MS/Quaternion Rotator2/Head to Limbic Angular Velocity Transform Rotation Matrix/Quaternion Integrator1 ==
  omega_limbic : Inport
  Demux1 : Demux
  Gain : Gain  Gain=1/delta_t
  Mux1 : Mux
  delta_q : Subsystem
  q0 : Integrator  InitialCondition=1
  q1 : Integrator
  q2 : Integrator
  q3 : Integrator
  q : Outport
  wires:
  Demux1/1 -> q0/1
  q0/1 -> Mux1/1
  Demux1/2 -> q1/1
  q1/1 -> Mux1/2
  Demux1/3 -> q2/1
  q2/1 -> Mux1/3
  Demux1/4 -> q3/1
  q3/1 -> Mux1/4
  Mux1/1 -> delta_q/2(q), q/1
  Gain/1 -> Demux1/1
  delta_q/1(delta_q) -> Gain/1
  omega_limbic/1 -> delta_q/1(omega)

== system observerModel_GVS_MS/Quaternion Rotator2/Head to Limbic Angular Velocity Transform Rotation Matrix/Quaternion to Direction Cosine1 ==
  note: A21
  q : Inport
  A1 : Subsystem
  A11 : Subsystem
  A12 : Subsystem
  A13 : Subsystem
  A22 : Subsystem
  A23 : Subsystem
  A31 : Subsystem
  A32 : Subsystem
  A33 : Subsystem
  Mux : Mux  Inputs=9
  Reshape (9) to [3x3] column-major : Reshape  OutputDimensionality=Customize  OutputDimensions=[3,3]
  D_Cos : Outport
  wires:
  A33/1(A33) -> Mux/9
  A32/1(A32) -> Mux/6
  A31/1(A31) -> Mux/3
  A23/1(A23) -> Mux/8
  A22/1(A22) -> Mux/5
  A13/1(A13) -> Mux/7
  A12/1(A12) -> Mux/4
  A11/1(A11) -> Mux/1
  q/1 -> A22/1(q), A1/1(q), A13/1(q), A12/1(q), A11/1(q), A23/1(q), A31/1(q), A32/1(q), A33/1(q)
  Reshape (9) to [3x3] column-major/1 -> D_Cos/1
  A1/1(A21) -> Mux/2
  Mux/1 -> Reshape (9) to [3x3] column-major/1

== system observerModel_GVS_MS/Quaternion Rotator2/Head to Limbic Angular Velocity Transform Rotation Matrix/Transform Axes ==
  limbic_cord : Inport
  Demux2 : Demux  Outputs=3
  Mux2 : Mux  Inputs=3
  VR_cord : Outport
  wires:
  limbic_cord/1 -> Demux2/1
  Mux2/1 -> VR_cord/1
  Demux2/3 -> Mux2/2
  Demux2/1 -> Mux2/3
  Demux2/2 -> Mux2/1

== system observerModel_GVS_MS/Quaternion Rotator2/Quaternion Integrator/delta_q ==
  omega : Inport
  q : Inport  Port=2
  C : Subsystem
  Constant : Constant  Value=delta_t
  K : Subsystem
  Product : Product  RndMeth=Zero
  Product1 : Product  RndMeth=Zero
  Product2 : Product  RndMeth=Zero
  Sum : Sum
  Z : Subsystem
  delta_q : Outport
  wires:
  q/1 -> C/2(q), Z/1(q), Product1/1
  Z/1(z) -> Product/1
  Product/1 -> Product1/2
  Product1/1 -> Sum/2
  C/1(C) -> Sum/1
  Sum/1 -> Product2/2
  Constant/1 -> Product2/1
  omega/1 -> C/1(omega)
  Product2/1 -> delta_q/1
  K/1(K) -> Product/2

== system observerModel_GVS_MS/Quaternion Rotator2/Quaternion to Direction Cosine/A1 ==
  q : Inport
  Demux : Demux
  Gain : Gain  Gain=2
  Product : Product  RndMeth=Zero
  Product1 : Product  RndMeth=Zero
  Sum : Sum  Inputs=+-
  A21 : Outport
  wires:
  q/1 -> Demux/1
  Sum/1 -> Gain/1
  Gain/1 -> A21/1
  Product/1 -> Sum/1
  Product1/1 -> Sum/2
  Demux/2 -> Product/1
  Demux/3 -> Product/2
  Demux/1 -> Product1/1
  Demux/4 -> Product1/2

== system observerModel_GVS_MS/Quaternion Rotator2/Quaternion to Direction Cosine/A11 ==
  q : Inport
  Demux : Demux
  Product{,1..3} (4 alike) : Product  RndMeth=Zero
  Sum : Sum  Inputs=++--
  A11 : Outport
  wires:
  Demux/1 -> Product/1, Product/2
  Demux/2 -> Product1/1, Product1/2
  Demux/3 -> Product2/1, Product2/2
  Demux/4 -> Product3/1, Product3/2
  Product/1 -> Sum/1
  Product1/1 -> Sum/2
  Product2/1 -> Sum/3
  Product3/1 -> Sum/4
  q/1 -> Demux/1
  Sum/1 -> A11/1

== system observerModel_GVS_MS/Quaternion Rotator2/Quaternion to Direction Cosine/A12 ==
  q : Inport
  Demux : Demux
  Gain : Gain  Gain=2
  Product : Product  RndMeth=Zero
  Product1 : Product  RndMeth=Zero
  Sum : Sum
  A12 : Outport
  wires:
  q/1 -> Demux/1
  Sum/1 -> Gain/1
  Gain/1 -> A12/1
  Demux/2 -> Product/1
  Demux/3 -> Product/2
  Demux/1 -> Product1/1
  Demux/4 -> Product1/2
  Product/1 -> Sum/1
  Product1/1 -> Sum/2

== system observerModel_GVS_MS/Quaternion Rotator2/Quaternion to Direction Cosine/A13 ==
  q : Inport
  Demux : Demux
  Gain : Gain  Gain=2
  Product : Product  RndMeth=Zero
  Product1 : Product  RndMeth=Zero
  Sum : Sum  Inputs=+-
  A13 : Outport
  wires:
  q/1 -> Demux/1
  Sum/1 -> Gain/1
  Gain/1 -> A13/1
  Product/1 -> Sum/1
  Product1/1 -> Sum/2
  Demux/2 -> Product/1
  Demux/4 -> Product/2
  Demux/1 -> Product1/1
  Demux/3 -> Product1/2

== system observerModel_GVS_MS/Quaternion Rotator2/Quaternion to Direction Cosine/A22 ==
  q : Inport
  Demux : Demux
  Product{,1..3} (4 alike) : Product  RndMeth=Zero
  Sum : Sum  Inputs=+-+-
  A22 : Outport
  wires:
  Demux/1 -> Product/1, Product/2
  Demux/2 -> Product1/1, Product1/2
  Demux/3 -> Product2/1, Product2/2
  Demux/4 -> Product3/1, Product3/2
  Product/1 -> Sum/1
  Product1/1 -> Sum/2
  Product2/1 -> Sum/3
  Product3/1 -> Sum/4
  q/1 -> Demux/1
  Sum/1 -> A22/1

== system observerModel_GVS_MS/Quaternion Rotator2/Quaternion to Direction Cosine/A23 ==
  q : Inport
  Demux : Demux
  Gain : Gain  Gain=2
  Product : Product  RndMeth=Zero
  Product1 : Product  RndMeth=Zero
  Sum : Sum
  A23 : Outport
  wires:
  q/1 -> Demux/1
  Sum/1 -> Gain/1
  Gain/1 -> A23/1
  Product/1 -> Sum/1
  Product1/1 -> Sum/2
  Demux/3 -> Product1/1
  Demux/4 -> Product1/2
  Demux/1 -> Product/1
  Demux/2 -> Product/2

== system observerModel_GVS_MS/Quaternion Rotator2/Quaternion to Direction Cosine/A31 ==
  q : Inport
  Demux : Demux
  Gain : Gain  Gain=2
  Product : Product  RndMeth=Zero
  Product1 : Product  RndMeth=Zero
  Sum : Sum
  A31 : Outport
  wires:
  q/1 -> Demux/1
  Sum/1 -> Gain/1
  Gain/1 -> A31/1
  Product/1 -> Sum/1
  Product1/1 -> Sum/2
  Demux/1 -> Product/1
  Demux/3 -> Product/2
  Demux/2 -> Product1/1
  Demux/4 -> Product1/2

== system observerModel_GVS_MS/Quaternion Rotator2/Quaternion to Direction Cosine/A32 ==
  q : Inport
  Demux : Demux
  Gain : Gain  Gain=2
  Product : Product  RndMeth=Zero
  Product1 : Product  RndMeth=Zero
  Sum : Sum  Inputs=+-
  A32 : Outport
  wires:
  q/1 -> Demux/1
  Sum/1 -> Gain/1
  Gain/1 -> A32/1
  Product/1 -> Sum/1
  Product1/1 -> Sum/2
  Demux/3 -> Product/1
  Demux/4 -> Product/2
  Demux/1 -> Product1/1
  Demux/2 -> Product1/2

== system observerModel_GVS_MS/Quaternion Rotator2/Quaternion to Direction Cosine/A33 ==
  q : Inport
  Demux : Demux
  Product{,1..3} (4 alike) : Product  RndMeth=Zero
  Sum : Sum  Inputs=+--+
  A33 : Outport
  wires:
  Demux/1 -> Product/1, Product/2
  Demux/2 -> Product1/1, Product1/2
  Demux/3 -> Product2/1, Product2/2
  Demux/4 -> Product3/1, Product3/2
  Product/1 -> Sum/1
  Product1/1 -> Sum/2
  Product2/1 -> Sum/3
  Product3/1 -> Sum/4
  q/1 -> Demux/1
  Sum/1 -> A33/1

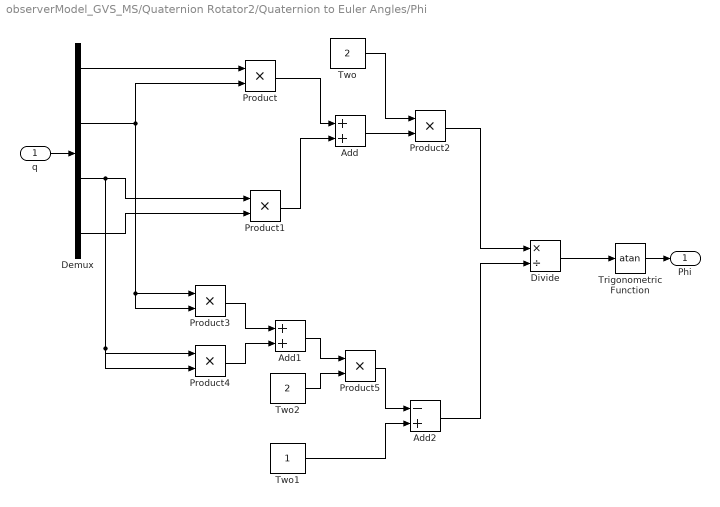
== system observerModel_GVS_MS/Quaternion Rotator2/Quaternion to Euler Angles/Phi ==
  q : Inport
  Add : Sum
  Add1 : Sum
  Add2 : Sum  Inputs=-+
  Demux : Demux
  Divide : Product  Inputs=*/
  Product{,1..5} (6 alike) : Product  RndMeth=Zero
  Trigonometric Function : Trigonometry  Operator=atan
  Two : Constant  Value=2  VectorParams1D=off
  Two1 : Constant  VectorParams1D=off
  Two2 : Constant  Value=2  VectorParams1D=off
  Phi : Outport
  wires:
  Demux/1 -> Product/1
  Demux/2 -> Product/2, Product3/1, Product3/2
  Product/1 -> Add/1
  Demux/4 -> Product1/2
  Demux/3 -> Product1/1, Product4/1, Product4/2
  Product1/1 -> Add/2
  Add/1 -> Product2/2
  Two/1 -> Product2/1
  Product3/1 -> Add1/1
  Product4/1 -> Add1/2
  Add1/1 -> Product5/1
  Two2/1 -> Product5/2
  Product5/1 -> Add2/1
  Two1/1 -> Add2/2
  Product2/1 -> Divide/1
  Add2/1 -> Divide/2
  Divide/1 -> Trigonometric Function/1
  q/1 -> Demux/1
  Trigonometric Function/1 -> Phi/1

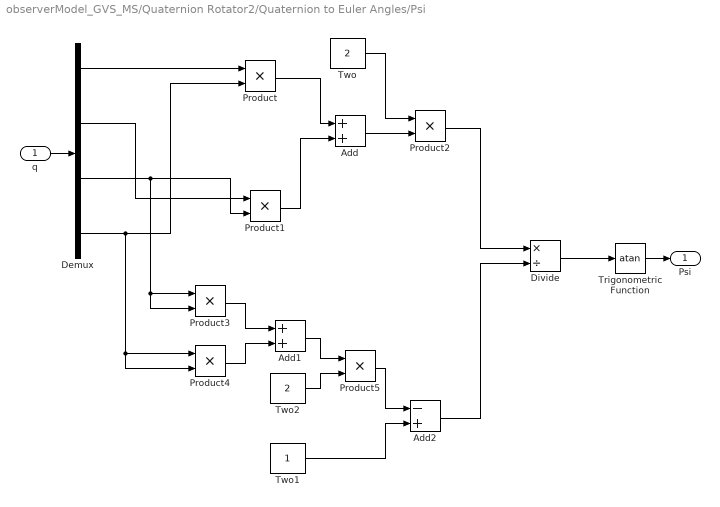
== system observerModel_GVS_MS/Quaternion Rotator2/Quaternion to Euler Angles/Psi ==
  q : Inport
  Add : Sum
  Add1 : Sum
  Add2 : Sum  Inputs=-+
  Demux : Demux
  Divide : Product  Inputs=*/
  Product{,1..5} (6 alike) : Product  RndMeth=Zero
  Trigonometric Function : Trigonometry  Operator=atan
  Two : Constant  Value=2  VectorParams1D=off
  Two1 : Constant  VectorParams1D=off
  Two2 : Constant  Value=2  VectorParams1D=off
  Psi : Outport
  wires:
  Demux/2 -> Product1/1
  Product/1 -> Add/1
  Demux/4 -> Product4/1, Product4/2, Product/2
  Product1/1 -> Add/2
  Add/1 -> Product2/2
  Two/1 -> Product2/1
  Product3/1 -> Add1/1
  Product4/1 -> Add1/2
  Add1/1 -> Product5/1
  Two2/1 -> Product5/2
  Product5/1 -> Add2/1
  Two1/1 -> Add2/2
  Product2/1 -> Divide/1
  Add2/1 -> Divide/2
  Divide/1 -> Trigonometric Function/1
  q/1 -> Demux/1
  Trigonometric Function/1 -> Psi/1
  Demux/1 -> Product/1
  Demux/3 -> Product1/2, Product3/1, Product3/2

== system observerModel_GVS_MS/Quaternion Rotator2/Quaternion to Euler Angles/Theta ==
  q : Inport
  Add : Sum  Inputs=+-
  Demux : Demux
  Product : Product  RndMeth=Zero
  Product1 : Product  RndMeth=Zero
  Product2 : Product  RndMeth=Zero
  Trigonometric Function : Trigonometry  Operator=asin
  Two : Constant  Value=2  VectorParams1D=off
  Theta : Outport
  wires:
  Demux/1 -> Product/1
  Product/1 -> Add/1
  Demux/4 -> Product1/2
  Product1/1 -> Add/2
  Add/1 -> Product2/2
  Two/1 -> Product2/1
  q/1 -> Demux/1
  Trigonometric Function/1 -> Theta/1
  Product2/1 -> Trigonometric Function/1
  Demux/3 -> Product/2
  Demux/2 -> Product1/1

== system observerModel_GVS_MS/Quaternion Rotator2/Rotation/Azimuthal Integrator ==
  g : Inport
  D_Cos : Inport  Port=2
  omega_rad : Inport  Port=3
  Dot Product : DotProduct  OutDataTypeStr=Inherit: Inherit via internal rule
  Gain : Gain  Gain=180/3.14159
  Integrator : Integrator
  Matrix Multiplication1 : Subsystem
  Scope1 : Scope
  azimuth : Outport
  wires:
  Matrix Multiplication1/1(omega_rad') -> Dot Product/2
  Dot Product/1 -> Gain/1, Integrator/1
  Gain/1 -> Scope1/1
  Integrator/1 -> azimuth/1
  g/1 -> Dot Product/1
  D_Cos/1 -> Matrix Multiplication1/1(D_Cos)
  omega_rad/1 -> Matrix Multiplication1/2(omega_rad)

== system observerModel_GVS_MS/Quaternion Rotator2/Rotation/Matrix Multiplication ==
  D_Cos : Inport
  GG0 : Inport  Port=2
  Demux : Demux  Outputs=3
      settings: DisplayOption=none
  Mux : Mux  Inputs=3
  Product : Product  Multiplication=Matrix(*)  RndMeth=Zero
  g : Outport
  wires:
  Product/1 -> Demux/1
  Demux/1 -> Mux/1
  Demux/2 -> Mux/2
  Demux/3 -> Mux/3
  D_Cos/1 -> Product/1
  Mux/1 -> g/1
  GG0/1 -> Product/2

== system observerModel_GVS_MS/Quaternion Rotator2/Tilt & SVV/SVV Calculator ==
  g : Inport
  Demux : Demux  Outputs=3
  Divide : Product  Inputs=*/
  Terminator : Terminator
  Trigonometric Function : Trigonometry  Operator=atan
  SVV : Outport
  wires:
  Divide/1 -> Trigonometric Function/1
  g/1 -> Demux/1
  Trigonometric Function/1 -> SVV/1
  Demux/2 -> Divide/1
  Demux/3 -> Divide/2
  Demux/1 -> Terminator/1

== system observerModel_GVS_MS/Quaternion Rotator2/Tilt & SVV/Tilt Calculator ==
  g : Inport
  Add : Sum  Inputs=+++
  Demux : Demux  Outputs=3
  Divide : Product  Inputs=*/
  Math Function : Math  Operator=sqrt  SignedPower=on
  Product{,1..3} (4 alike) : Product  RndMeth=Zero
  Trigonometric Function : Trigonometry  Operator=acos  OutputSignalType=real
  Two : Constant  Value=-1  VectorParams1D=off
  Tilt : Outport
  wires:
  Product/1 -> Add/1
  Product1/1 -> Add/2
  Divide/1 -> Trigonometric Function/1
  g/1 -> Demux/1
  Product2/1 -> Add/3
  Demux/1 -> Product/1, Product/2
  Demux/2 -> Product1/2, Product1/1
  Demux/3 -> Product2/2, Product2/1, Product3/1
  Add/1 -> Math Function/1
  Two/1 -> Product3/2
  Math Function/1 -> Divide/2
  Product3/1 -> Divide/1
  Trigonometric Function/1 -> Tilt/1

== system observerModel_GVS_MS/SCC GVS /Left Irregular Hyper//Depol /If Action Subsystem ==
  In1 : Inport
  Action Port : ActionPort  ActionPortLabel=if(u1 > 0)
  Transfer Fcn1 : TransferFcn  Numerator=IrregSCC2Physical.Numerator{1,1}  Denominator=IrregSCC2Physical.Denominator{1,1}
  Transfer Fcn2 : TransferFcn  Numerator=IrregHyperpol.Numerator{1,1}  Denominator=IrregHyperpol.Denominator{1,1}
  Out1 : Outport
  wires:
  Transfer Fcn1/1 -> Out1/1
  In1/1 -> Transfer Fcn2/1
  Transfer Fcn2/1 -> Transfer Fcn1/1

== system observerModel_GVS_MS/SCC GVS /Left Irregular Hyper//Depol /If Action Subsystem1 ==
  In1 : Inport
  Action Port : ActionPort  ActionPortLabel=else
  Transfer Fcn1 : TransferFcn  Numerator=IrregSCC2Physical.Numerator{1,1}  Denominator=IrregSCC2Physical.Denominator{1,1}
  Transfer Fcn2 : TransferFcn  Numerator=IrregDepol.Numerator{1,1}  Denominator=IrregDepol.Denominator{1,1}
  Out1 : Outport
  wires:
  Transfer Fcn1/1 -> Out1/1
  In1/1 -> Transfer Fcn2/1
  Transfer Fcn2/1 -> Transfer Fcn1/1

== system observerModel_GVS_MS/SCC GVS /Left Regular Hyper//Depol/If Action Subsystem ==
  In1 : Inport
  Action Port : ActionPort  ActionPortLabel=if(u1 > 0)
  Transfer Fcn1 : TransferFcn  Numerator=RegSCC2Physical.Numerator{1,1}  Denominator=RegSCC2Physical.Denominator{1,1}
  Transfer Fcn2 : TransferFcn  Numerator=RegHyperpol.Numerator{1,1}  Denominator=RegHyperpol.Denominator{1,1}
  Out1 : Outport
  wires:
  In1/1 -> Transfer Fcn2/1
  Transfer Fcn2/1 -> Transfer Fcn1/1
  Transfer Fcn1/1 -> Out1/1

== system observerModel_GVS_MS/SCC GVS /Left Regular Hyper//Depol/If Action Subsystem1 ==
  In1 : Inport
  Action Port : ActionPort  ActionPortLabel=else
  Transfer Fcn1 : TransferFcn  Numerator=RegSCC2Physical.Numerator{1,1}  Denominator=RegSCC2Physical.Denominator{1,1}
  Transfer Fcn2 : TransferFcn  Numerator=RegDepol.Numerator{1,1}  Denominator=RegDepol.Denominator{1,1}
  Out1 : Outport
  wires:
  In1/1 -> Transfer Fcn2/1
  Transfer Fcn2/1 -> Transfer Fcn1/1
  Transfer Fcn1/1 -> Out1/1

== system observerModel_GVS_MS/SCC GVS /Right Irregular Hyper//Depol /If Action Subsystem ==
  In1 : Inport
  Action Port : ActionPort  ActionPortLabel=if(u1 > 0)
  Transfer Fcn1 : TransferFcn  Numerator=IrregSCC2Physical.Numerator{1,1}  Denominator=IrregSCC2Physical.Denominator{1,1}
  Transfer Fcn2 : TransferFcn  Numerator=IrregHyperpol.Numerator{1,1}  Denominator=IrregHyperpol.Denominator{1,1}
  Out1 : Outport
  wires:
  Transfer Fcn1/1 -> Out1/1
  In1/1 -> Transfer Fcn2/1
  Transfer Fcn2/1 -> Transfer Fcn1/1

== system observerModel_GVS_MS/SCC GVS /Right Irregular Hyper//Depol /If Action Subsystem1 ==
  In1 : Inport
  Action Port : ActionPort  ActionPortLabel=else
  Transfer Fcn1 : TransferFcn  Numerator=IrregSCC2Physical.Numerator{1,1}  Denominator=IrregSCC2Physical.Denominator{1,1}
  Transfer Fcn2 : TransferFcn  Numerator=IrregDepol.Numerator{1,1}  Denominator=IrregDepol.Denominator{1,1}
  Out1 : Outport
  wires:
  Transfer Fcn1/1 -> Out1/1
  In1/1 -> Transfer Fcn2/1
  Transfer Fcn2/1 -> Transfer Fcn1/1

== system observerModel_GVS_MS/SCC GVS /Right Regular Hyper//Depol /If Action Subsystem ==
  In1 : Inport
  Action Port : ActionPort  ActionPortLabel=if(u1 > 0)
  Transfer Fcn1 : TransferFcn  Numerator=RegSCC2Physical.Numerator{1,1}  Denominator=RegSCC2Physical.Denominator{1,1}
  Transfer Fcn2 : TransferFcn  Numerator=RegHyperpol.Numerator{1,1}  Denominator=RegHyperpol.Denominator{1,1}
  Out1 : Outport
  wires:
  Transfer Fcn1/1 -> Out1/1
  In1/1 -> Transfer Fcn2/1
  Transfer Fcn2/1 -> Transfer Fcn1/1

== system observerModel_GVS_MS/SCC GVS /Right Regular Hyper//Depol /If Action Subsystem1 ==
  In1 : Inport
  Action Port : ActionPort  ActionPortLabel=else
  Transfer Fcn1 : TransferFcn  Numerator=RegSCC2Physical.Numerator{1,1}  Denominator=RegSCC2Physical.Denominator{1,1}
  Transfer Fcn2 : TransferFcn  Numerator=RegDepol.Numerator{1,1}  Denominator=RegDepol.Denominator{1,1}
  Out1 : Outport
  wires:
  In1/1 -> Transfer Fcn2/1
  Transfer Fcn2/1 -> Transfer Fcn1/1
  Transfer Fcn1/1 -> Out1/1

== system observerModel_GVS_MS/Subsystem3/Subsystem3/Matrix Multiplication ==
  D_Cos : Inport
  a_world : Inport  Port=2
  Demux : Demux  Outputs=3
      settings: DisplayOption=none
  Mux : Mux  Inputs=3
  Product : Product  Multiplication=Matrix(*)  RndMeth=Zero
  a_head : Outport
  wires:
  Product/1 -> Demux/1
  Demux/1 -> Mux/1
  Demux/2 -> Mux/2
  Demux/3 -> Mux/3
  D_Cos/1 -> Product/1
  Mux/1 -> a_head/1
  a_world/1 -> Product/2

== system observerModel_GVS_MS/Subsystem3/Subsystem4/Matrix Multiplication ==
  D_Cos : Inport
  a_esr_head : Inport  Port=2
  Demux : Demux  Outputs=3
      settings: DisplayOption=none
  Math Function : Math  Operator=transpose  SignedPower=on
  Mux : Mux  Inputs=3
  Product : Product  Multiplication=Matrix(*)  RndMeth=Zero
  a_est_world : Outport
  wires:
  Product/1 -> Demux/1
  Demux/1 -> Mux/1
  Demux/2 -> Mux/2
  Demux/3 -> Mux/3
  D_Cos/1 -> Math Function/1
  Mux/1 -> a_est_world/1
  a_esr_head/1 -> Product/2
  Math Function/1 -> Product/1

== system observerModel_GVS_MS/Subsystem5/Subsystem3/Matrix Multiplication ==
  D_Cos : Inport
  a_world : Inport  Port=2
  Demux : Demux  Outputs=3
      settings: DisplayOption=none
  Mux : Mux  Inputs=3
  Product : Product  Multiplication=Matrix(*)  RndMeth=Zero
  a_head : Outport
  wires:
  Product/1 -> Demux/1
  Demux/1 -> Mux/1
  Demux/2 -> Mux/2
  Demux/3 -> Mux/3
  D_Cos/1 -> Product/1
  Mux/1 -> a_head/1
  a_world/1 -> Product/2
